simulink model "pendulo_invertidoOF"  (R2026a)
settings: Solver=VariableStepAuto
InitFcn:
  | Ip = 0.0079;
  | Mc = 0.7031;
  | lp = 0.3302;
  | Mp = 0.23;
  | Beq = 4.3;
  | g = 9.81;
  | Bp = 0.0024;
  | Fc = 0;
settings Model: Creator=elmik  LastModifiedBy=elmik

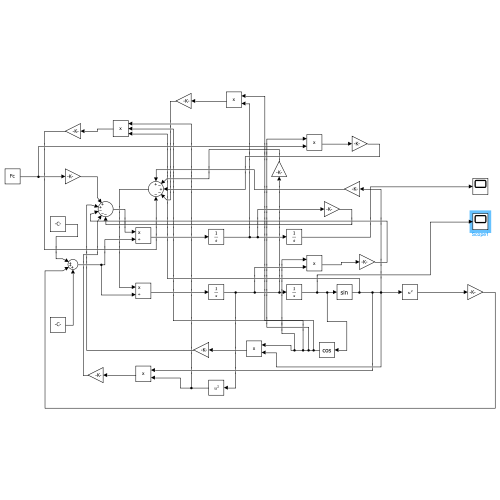
[thumbnail: Simulink's stored preview of the top-level diagram]
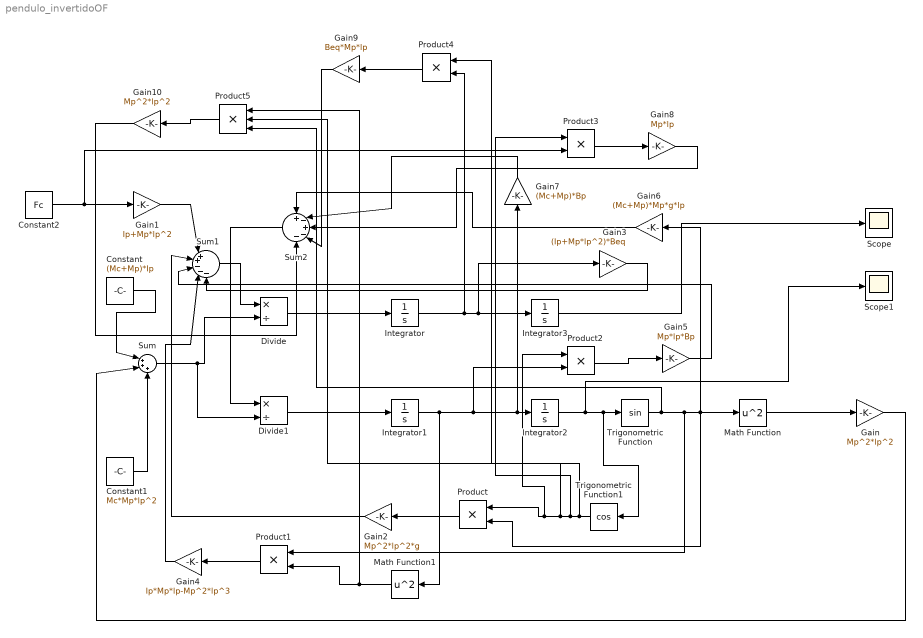
== system pendulo_invertidoOF ==
  Constant : Constant  Value=(Mc+Mp)*Ip
  Constant1 : Constant  Value=Mc*Mp*lp^2
  Constant2 : Constant  Value=Fc
  Divide : Product  Inputs=*/
  Divide1 : Product  Inputs=*/
  Gain : Gain  Gain=Mp^2*lp^2
  Gain1 : Gain  Gain=Ip+Mp*lp^2
  Gain10 : Gain  Gain=Mp^2*lp^2
  Gain2 : Gain  Gain=Mp^2*lp^2*g
  Gain3 : Gain  Gain=(Ip+Mp*lp^2)*Beq
  Gain4 : Gain  Gain=Ip*Mp*lp-Mp^2*lp^3
  Gain5 : Gain  Gain=Mp*lp*Bp
  Gain6 : Gain  Gain=(Mc+Mp)*Mp*g*lp
  Gain7 : Gain  Gain=(Mc+Mp)*Bp
  Gain8 : Gain  Gain=Mp*lp
  Gain9 : Gain  Gain=Beq*Mp*lp
  Integrator : Integrator
  Integrator1 : Integrator
  Integrator2 : Integrator  InitialCondition=pi/180
  Integrator3 : Integrator
  Math Function : Math  Operator=square
  Math Function1 : Math  Operator=square
  Product{,1..4} (5 alike) : Product
  Product5 : Product  Inputs=3
  Scope : Scope
      settings: ActiveDisplayYMinimum=-0.025100764837812897  ActiveDisplayYMaximum=0.22590688354031613
  Scope1 : Scope
      settings: ActiveDisplayYMinimum=-12.296569831702669  ActiveDisplayYMaximum=110.84366141052348
  Sum : Sum  Inputs=|+++
  Sum1 : Sum  Inputs=|++---
  Sum2 : Sum  Inputs=+-+--
  Trigonometric Function : Trigonometry
  Trigonometric Function1 : Trigonometry  Operator=cos
  wires:
  Divide/1 -> Integrator/1
  Divide1/1 -> Integrator1/1
  Sum/1 -> Divide1/2, Divide/2
  Constant/1 -> Sum/1
  Constant1/1 -> Sum/3
  Integrator2/1 -> Scope1/1, Trigonometric Function/1, Trigonometric Function1/1
  Trigonometric Function/1 -> Product5/3, Gain6/1, Product/2, Math Function/1, Product1/1
  Math Function/1 -> Gain/1
  Gain/1 -> Sum/2
  Integrator/1 -> Product4/2, Gain3/1, Integrator3/1
  Integrator1/1 -> Product2/2, Gain7/1, Integrator2/1, Math Function1/1
  Sum1/1 -> Divide/1
  Gain1/1 -> Sum1/1
  Constant2/1 -> Product3/2, Gain1/1
  Trigonometric Function1/1 -> Product5/2, Product3/1, Product4/1, Product2/1, Product/1
  Product/1 -> Gain2/1
  Gain3/1 -> Sum1/5
  Math Function1/1 -> Product5/1, Product1/2
  Product1/1 -> Gain4/1
  Gain4/1 -> Sum1/4
  Product2/1 -> Gain5/1
  Gain5/1 -> Sum1/3
  Gain2/1 -> Sum1/2
  Sum2/1 -> Divide1/1
  Gain6/1 -> Sum2/1
  Gain7/1 -> Sum2/2
  Product3/1 -> Gain8/1
  Gain8/1 -> Sum2/3
  Product4/1 -> Gain9/1
  Gain9/1 -> Sum2/4
  Gain10/1 -> Sum2/5
  Product5/1 -> Gain10/1
  Integrator3/1 -> Scope/1
